simulink model "liniowy_model_z_przesunieciami"  (R2017a)
settings: Solver=ode45  StartTime=0.0  StopTime=40  MaxStep=0.0001  RelTol=1e-5  EnableMultiTasking=on
values from neighbouring files (symbols this model uses):
  A = [0 0 1 0]    [Linearyzacja_ramienia_robota.m]    (also in model_nie_liniowy.m = [0 0 1 0; sciaga.m; zad1.m = double(A); zad1_v3.m = double(A))
  B = [0 0; 0 0; double(d1); double(d2)]    [Linearyzacja_ramienia_robota.m]    (also in model_nie_liniowy.m = [0 0; sciaga.m; zad1.m = [0 0; zad1_v3.m = [0 0)
  L = lqr(A, B, Q, R)    [Linearyzacja_ramienia_robota.m]    (also in filtr_kalmana_Mateusz.m = (eye(4) - K*C_D)*B_D; sciaga.m = lqr(A,B,Q,R))
settings Model: Creator=kss  LastModifiedBy=Szwank
settings OptimizationCC: LifeSpan=inf
settings DebuggingCC: SFUnexpectedBacktrackingDiag=warning  SFNoUnconditionalDefaultTransitionDiag=warning  SFExecutionAtInitializationDiag=none
settings GRTTargetCC: TargetLangStandard=C89/C90 (ANSI)  GeneratePreprocessorConditionals=Disable all
settings ConfigComp: CovMetricSettings=dw  CovHtmlReporting=on  CovSaveCumulativeToWorkspaceVar=on  CovSaveSingleToWorkspaceVar=on  CovExternalEMLEnable=off

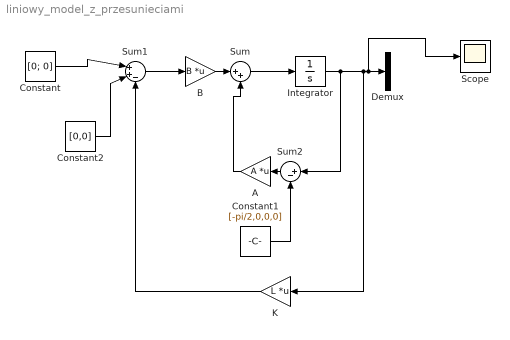
== system liniowy_model_z_przesunieciami ==
  A : Gain  Gain=A  Multiplication=Matrix(K*u)
  B : Gain  Gain=B  Multiplication=Matrix(K*u)
  Constant : Constant  Value=[0; 0]
  Constant1 : Constant  Value=[-pi/2,0,0,0]
  Constant2 : Constant  Value=[0,0]
  Demux : Demux
  Integrator : Integrator  InitialCondition=[pi/2,0,0,0]
  K : Gain  Gain=L  Multiplication=Matrix(K*u)
  Scope : Scope
  Sum : Sum  Inputs=|++
  Sum1 : Sum  Inputs=|++-
  Sum2 : Sum  Inputs=|+-
  wires:
  Integrator/1 -> Sum2/1, K/1, Scope/1, Demux/1
  A/1 -> Sum/2
  Sum/1 -> Integrator/1
  B/1 -> Sum/1
  Sum2/1 -> A/1
  Sum1/1 -> B/1
  Constant2/1 -> Sum1/2
  Constant/1 -> Sum1/1
  K/1 -> Sum1/3
  Constant1/1 -> Sum2/2
